simulink model "mdlRef"  (R2023b)
settings: Solver=VariableStepAuto  StartTime=0.0  StopTime=10.0  RelTol=1e-3
settings Model: Creator=neham  LastModifiedBy=neham

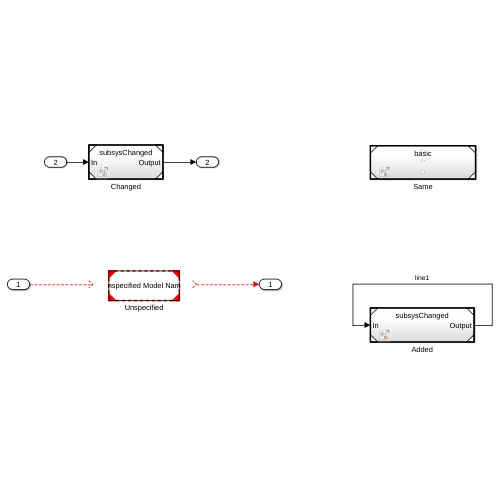
[thumbnail: Simulink's stored preview of the top-level diagram]
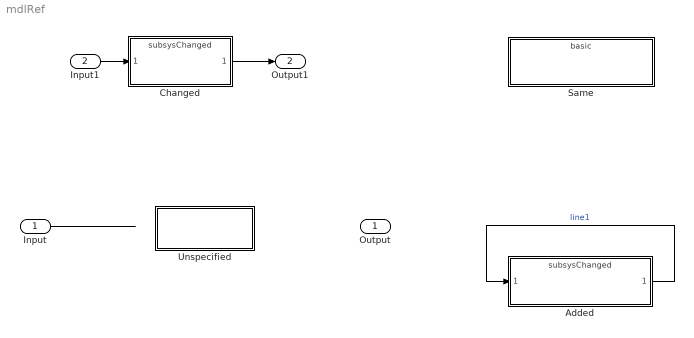
== system mdlRef ==
  Input : Inport
  Input1 : Inport  Port=2
  Added : ModelReference  ModelNameDialog=subsysChanged.slx  SimulationMode=Normal  ModelReferenceVersion=1.1
  Changed : ModelReference  ModelNameDialog=subsysChanged.slx  SimulationMode=Normal  ModelReferenceVersion=1.1
  Same : ModelReference  ModelNameDialog=basic.slx  SimulationMode=Normal  ModelReferenceVersion=1.4
  Unspecified : ModelReference  SimulationMode=Normal
  Output : Outport
  Output1 : Outport  Port=2
  wires:
  Input/1 -> ?
  ? -> Output/1
  Input1/1 -> Changed/1
  Changed/1 -> Output1/1
  Added/1 -> Added/1  "line1"
